simulink model "hexapod2"  (R2015a)
settings: Solver=ode23tb  StartTime=0.0  StopTime=10  FixedStep=0.0001  MaxStep=0.01  RelTol=1e-4  AbsTol=1e-5
values from neighbouring files (symbols this model uses):
  bH = 1    [runFirst.m]
  C = CM + CL/n^2    (= 0.0001377500155)    [runFirst.m]
  d1 = 0    [runFirst.m]    (also in runFirst2.m)
  d2 = -4.61    [runFirst.m]    (also in runFirst2.m = 0)
  J = JM + JL/n^2    (= 0.008455500031)    [runFirst.m]
  Ka = 12    [runFirst.m]
  Kb = 0.00867    [runFirst.m]
  Ke = 1    [runFirst.m]
  Km = 4.375    [runFirst.m]
  L = 0.0006    [runFirst.m]
  L1 = 3.64    [runFirst.m]    (also in runFirst2.m = 3.4)
  L2 = 5.72    [runFirst.m]    (also in runFirst2.m = 8.7)
  L3 = 12.46    [runFirst.m]    (also in runFirst2.m = 12.73)
  n = 254    [runFirst.m]
  R = 1.4    [runFirst.m]
undefined symbols (not defined in the file or in its folder): bLb, bLs, X, Y, Z
libraries: sm_lib x108, nesl_utility x43, simulink x24, Contact_Forces_Lib x7, roblocks x2
(part 4 of 5)

== system hexapod2/Hexapod/Leg4/Link3 ==
  Reference Frame : sm_lib/Frames and Transforms/Reference Frame  BlockFunction=simmechanics.library.frames_transforms.reference_frame
  Rigid Transform : sm_lib/Frames and Transforms/Rigid Transform  TranslationMethod=StandardAxis  TranslationLengthUnit=cm  TranslationStandardAxis=+X  TranslationStandardOffset=L/2  TranslationCartesianOffset=[0 0 0]  TranslationROffset=0  TranslationROffsetUnits=m  TranslationZOffset=0  TranslationZOffsetUnits=m  TranslationThetaOffset=0  TranslationThetaOffsetUnits=deg  RotationMethod=None  RotationAngleUnits=deg  RotationStandardAxis=+X  RotationAngle=Xangle  RotationArbitraryAxis=[0 0 1]  FollAlignAxisA=+X  BaseAlignAxisA=+Y  FollAlignAxisB=+Y  BaseAlignAxisB=+Z  RotationMatrix=[1 0 0; 0 1 0; 0 0 1]  BlockFunction=simmechanics.library.frames_transforms.rigid_transform
  Rigid Transform1 : sm_lib/Frames and Transforms/Rigid Transform  TranslationMethod=StandardAxis  TranslationLengthUnit=cm  TranslationStandardAxis=-X  TranslationStandardOffset=L/2  TranslationCartesianOffset=[0 0 0]  TranslationROffset=0  TranslationROffsetUnits=m  TranslationZOffset=0  TranslationZOffsetUnits=m  TranslationThetaOffset=0  TranslationThetaOffsetUnits=deg  RotationMethod=None  RotationAngleUnits=deg  RotationStandardAxis=+Z  RotationAngle=0.0  RotationArbitraryAxis=[0 0 1]  FollAlignAxisA=+X  BaseAlignAxisA=+Y  FollAlignAxisB=+Y  BaseAlignAxisB=+Z  RotationMatrix=[1 0 0; 0 1 0; 0 0 1]  BlockFunction=simmechanics.library.frames_transforms.rigid_transform
  Solid : sm_lib/Body Elements/Solid  InertiaType=PointMass  Mass=m  MassUnits=kg  CenterOfMass=[0 0 0]  CenterOfMassUnits=m  MomentsOfInertia=[1 1 1]  MomentsOfInertiaUnits=kg*m^2  ProductsOfInertia=[0 0 0]  ProductsOfInertiaUnits=kg*m^2  DensityBased=off  Density=1  DensityUnits=kg/(m^3)  GraphicType=FromGeometry  MarkerShape=Sphere  MarkerSize=10  MarkerSizeUnits=m  GraphicVisPropType=SimpleVisualProperties  GraphicDiffuseColor=rgb  GraphicSpecularColor=[0.5 0.5 0.5 1.0]  GraphicAmbientColor=[0.15 0.15 0.15 1.0]  GraphicEmissiveColor=[0.0 0.0 0.0 1.0]  GraphicShininess=75  GraphicOpacity=1.0  GeometryShape=Brick  RectangleSize=[1 1]  RectangleSizeUnits=m  BrickDimensions=[L W H]  BrickDimensionUnits=cm  CylinderRadius=1  CylinderRadiusUnits=m  CylinderLength=1  CylinderLengthUnits=m  SphereRadius=1  SphereRadiusUnits=m  EllipsoidRadii=[1 1 1]  EllipsoidRadiiUnits=m  ExtrusionCrossSection=[1 1; -1 1; -1 -1; 1 -1]  ExtrusionCrossSectionUnits=m  ExtrusionLength=1  ExtrusionLengthUnits=m  PolygonNumSides=3  PolygonOuterRadius=1  PolygonOuterRadiusUnits=m  ExtGeomFileType=STL  ExtGeomFileUnits=m  RevolutionCrossSection=[1 1; 1 -1; 2 -1; 2 1]  RevolutionCrossSectionUnits=m  RevolutionExtent=Full  RevolutionAngle=180  RevolutionAngleUnits=deg  BlockFunction=simmechanics.library.body_elements.solid
  Conn1 : PMIOPort  Port=1  Side=Left
  Conn2 : PMIOPort  Port=2  Side=Right
  connections:
  Reference Frame/RConn1 -- Solid/RConn1 -- Rigid Transform/LConn1 -- Rigid Transform1/LConn1
  Rigid Transform/RConn1 -- Conn2/RConn1
  Rigid Transform1/RConn1 -- Conn1/RConn1

== system hexapod2/Hexapod/Leg4/Servo ==
  note: ThetaRef
  note: e
  note: Vref
  thetaRef : Inport
  PID : Subsystem
  Sum : Sum  Inputs=|+-
  Thet : Scope
      settings: TimeRange=10  YMin=0  YMax=21
  w : Scope
      settings: SaveName=ScopeData2
  wd : Scope
      settings: SaveName=ScopeData3
  Двигатель : Subsystem
  Заданный угол : Gain
  Энкодер : Gain  Gain=Ke
  theta : Outport
  wires:
  thetaRef/1 -> Заданный угол/1
  Двигатель/3(Ускорение) -> wd/1
  PID/1(Out1) -> Двигатель/1(Заданный угол)
  Двигатель/1(Угол) -> Энкодер/1, Thet/1, theta/1
  Энкодер/1 -> Sum/2
  Sum/1 -> PID/1(In1)
  Заданный угол/1 -> Sum/1
  Двигатель/2(Скорость) -> w/1

== system hexapod2/Hexapod/Leg4/Servo1 ==
  note: Vref
  note: e
  note: ThetaRef
  thetaRef : Inport
  PID : Subsystem
  Sum : Sum  Inputs=|+-
  Thet : Scope
      settings: TimeRange=10  YMin=0  YMax=21
  w : Scope
      settings: SaveName=ScopeData2
  wd : Scope
      settings: SaveName=ScopeData3
  Двигатель : Subsystem
  Заданный угол : Gain
  Энкодер : Gain  Gain=Ke
  theta : Outport
  wires:
  Двигатель/2(Скорость) -> w/1
  Заданный угол/1 -> Sum/1
  Sum/1 -> PID/1(In1)
  Энкодер/1 -> Sum/2
  Двигатель/1(Угол) -> theta/1, Thet/1, Энкодер/1
  PID/1(Out1) -> Двигатель/1(Заданный угол)
  Двигатель/3(Ускорение) -> wd/1
  thetaRef/1 -> Заданный угол/1

== system hexapod2/Hexapod/Leg4/Servo2 ==
  note: ThetaRef
  note: e
  note: Vref
  thetaRef : Inport
  PID : Subsystem
  Sum : Sum  Inputs=|+-
  Thet : Scope
      settings: TimeRange=10  YMin=0  YMax=21
  w : Scope
      settings: SaveName=ScopeData2
  wd : Scope
      settings: SaveName=ScopeData3
  Двигатель : Subsystem
  Заданный угол : Gain
  Энкодер : Gain  Gain=Ke
  theta : Outport
  wires:
  thetaRef/1 -> Заданный угол/1
  Двигатель/3(Ускорение) -> wd/1
  PID/1(Out1) -> Двигатель/1(Заданный угол)
  Двигатель/1(Угол) -> Энкодер/1, Thet/1, theta/1
  Энкодер/1 -> Sum/2
  Sum/1 -> PID/1(In1)
  Заданный угол/1 -> Sum/1
  Двигатель/2(Скорость) -> w/1

== system hexapod2/Hexapod/Leg5/Link1 ==
  Reference Frame : sm_lib/Frames and Transforms/Reference Frame  BlockFunction=simmechanics.library.frames_transforms.reference_frame
  Rigid Transform : sm_lib/Frames and Transforms/Rigid Transform  TranslationMethod=Cartesian  TranslationLengthUnit=cm  TranslationStandardAxis=+X  TranslationStandardOffset=L/2  TranslationCartesianOffset=[L/2 0 -2.3]  TranslationROffset=0  TranslationROffsetUnits=m  TranslationZOffset=0  TranslationZOffsetUnits=m  TranslationThetaOffset=0  TranslationThetaOffsetUnits=deg  RotationMethod=StandardAxis  RotationAngleUnits=deg  RotationStandardAxis=+X  RotationAngle=Xangle  RotationArbitraryAxis=[0 0 1]  FollAlignAxisA=+X  BaseAlignAxisA=+Y  FollAlignAxisB=+Y  BaseAlignAxisB=+Z  RotationMatrix=[1 0 0; 0 1 0; 0 0 1]  BlockFunction=simmechanics.library.frames_transforms.rigid_transform
  Rigid Transform1 : sm_lib/Frames and Transforms/Rigid Transform  TranslationMethod=StandardAxis  TranslationLengthUnit=cm  TranslationStandardAxis=-X  TranslationStandardOffset=L/2  TranslationCartesianOffset=[0 0 0]  TranslationROffset=0  TranslationROffsetUnits=m  TranslationZOffset=0  TranslationZOffsetUnits=m  TranslationThetaOffset=0  TranslationThetaOffsetUnits=deg  RotationMethod=None  RotationAngleUnits=deg  RotationStandardAxis=+Z  RotationAngle=0.0  RotationArbitraryAxis=[0 0 1]  FollAlignAxisA=+X  BaseAlignAxisA=+Y  FollAlignAxisB=+Y  BaseAlignAxisB=+Z  RotationMatrix=[1 0 0; 0 1 0; 0 0 1]  BlockFunction=simmechanics.library.frames_transforms.rigid_transform
  Solid : sm_lib/Body Elements/Solid  InertiaType=PointMass  Mass=m  MassUnits=kg  CenterOfMass=[0 0 0]  CenterOfMassUnits=m  MomentsOfInertia=[1 1 1]  MomentsOfInertiaUnits=kg*m^2  ProductsOfInertia=[0 0 0]  ProductsOfInertiaUnits=kg*m^2  DensityBased=off  Density=1  DensityUnits=kg/(m^3)  GraphicType=FromGeometry  MarkerShape=Sphere  MarkerSize=10  MarkerSizeUnits=m  GraphicVisPropType=SimpleVisualProperties  GraphicDiffuseColor=rgb  GraphicSpecularColor=[0.5 0.5 0.5 1.0]  GraphicAmbientColor=[0.15 0.15 0.15 1.0]  GraphicEmissiveColor=[0.0 0.0 0.0 1.0]  GraphicShininess=75  GraphicOpacity=1.0  GeometryShape=Brick  RectangleSize=[1 1]  RectangleSizeUnits=m  BrickDimensions=[L W H]  BrickDimensionUnits=cm  CylinderRadius=1  CylinderRadiusUnits=m  CylinderLength=1  CylinderLengthUnits=m  SphereRadius=1  SphereRadiusUnits=m  EllipsoidRadii=[1 1 1]  EllipsoidRadiiUnits=m  ExtrusionCrossSection=[1 1; -1 1; -1 -1; 1 -1]  ExtrusionCrossSectionUnits=m  ExtrusionLength=1  ExtrusionLengthUnits=m  PolygonNumSides=3  PolygonOuterRadius=1  PolygonOuterRadiusUnits=m  ExtGeomFileType=STL  ExtGeomFileUnits=m  RevolutionCrossSection=[1 1; 1 -1; 2 -1; 2 1]  RevolutionCrossSectionUnits=m  RevolutionExtent=Full  RevolutionAngle=180  RevolutionAngleUnits=deg  BlockFunction=simmechanics.library.body_elements.solid
  Conn1 : PMIOPort  Port=1  Side=Left
  Conn2 : PMIOPort  Port=2  Side=Right
  connections:
  Rigid Transform1/RConn1 -- Conn1/RConn1
  Rigid Transform/RConn1 -- Conn2/RConn1
  Rigid Transform1/LConn1 -- Rigid Transform/LConn1 -- Solid/RConn1 -- Reference Frame/RConn1

== system hexapod2/Hexapod/Leg5/Link2 ==
  Reference Frame : sm_lib/Frames and Transforms/Reference Frame  BlockFunction=simmechanics.library.frames_transforms.reference_frame
  Rigid Transform : sm_lib/Frames and Transforms/Rigid Transform  TranslationMethod=StandardAxis  TranslationLengthUnit=cm  TranslationStandardAxis=+X  TranslationStandardOffset=L/2  TranslationCartesianOffset=[0 0 0]  TranslationROffset=0  TranslationROffsetUnits=m  TranslationZOffset=0  TranslationZOffsetUnits=m  TranslationThetaOffset=0  TranslationThetaOffsetUnits=deg  RotationMethod=StandardAxis  RotationAngleUnits=deg  RotationStandardAxis=+X  RotationAngle=Xangle  RotationArbitraryAxis=[0 0 1]  FollAlignAxisA=+X  BaseAlignAxisA=+Y  FollAlignAxisB=+Y  BaseAlignAxisB=+Z  RotationMatrix=[1 0 0; 0 1 0; 0 0 1]  BlockFunction=simmechanics.library.frames_transforms.rigid_transform
  Rigid Transform1 : sm_lib/Frames and Transforms/Rigid Transform  TranslationMethod=StandardAxis  TranslationLengthUnit=cm  TranslationStandardAxis=-X  TranslationStandardOffset=L/2  TranslationCartesianOffset=[0 0 0]  TranslationROffset=0  TranslationROffsetUnits=m  TranslationZOffset=0  TranslationZOffsetUnits=m  TranslationThetaOffset=0  TranslationThetaOffsetUnits=deg  RotationMethod=None  RotationAngleUnits=deg  RotationStandardAxis=+Z  RotationAngle=0.0  RotationArbitraryAxis=[0 0 1]  FollAlignAxisA=+X  BaseAlignAxisA=+Y  FollAlignAxisB=+Y  BaseAlignAxisB=+Z  RotationMatrix=[1 0 0; 0 1 0; 0 0 1]  BlockFunction=simmechanics.library.frames_transforms.rigid_transform
  Solid : sm_lib/Body Elements/Solid  InertiaType=PointMass  Mass=m  MassUnits=kg  CenterOfMass=[0 0 0]  CenterOfMassUnits=m  MomentsOfInertia=[1 1 1]  MomentsOfInertiaUnits=kg*m^2  ProductsOfInertia=[0 0 0]  ProductsOfInertiaUnits=kg*m^2  DensityBased=off  Density=1  DensityUnits=kg/(m^3)  GraphicType=FromGeometry  MarkerShape=Sphere  MarkerSize=10  MarkerSizeUnits=m  GraphicVisPropType=SimpleVisualProperties  GraphicDiffuseColor=rgb  GraphicSpecularColor=[0.5 0.5 0.5 1.0]  GraphicAmbientColor=[0.15 0.15 0.15 1.0]  GraphicEmissiveColor=[0.0 0.0 0.0 1.0]  GraphicShininess=75  GraphicOpacity=1.0  GeometryShape=Brick  RectangleSize=[1 1]  RectangleSizeUnits=m  BrickDimensions=[L W H]  BrickDimensionUnits=cm  CylinderRadius=1  CylinderRadiusUnits=m  CylinderLength=1  CylinderLengthUnits=m  SphereRadius=1  SphereRadiusUnits=m  EllipsoidRadii=[1 1 1]  EllipsoidRadiiUnits=m  ExtrusionCrossSection=[1 1; -1 1; -1 -1; 1 -1]  ExtrusionCrossSectionUnits=m  ExtrusionLength=1  ExtrusionLengthUnits=m  PolygonNumSides=3  PolygonOuterRadius=1  PolygonOuterRadiusUnits=m  ExtGeomFileType=STL  ExtGeomFileUnits=m  RevolutionCrossSection=[1 1; 1 -1; 2 -1; 2 1]  RevolutionCrossSectionUnits=m  RevolutionExtent=Full  RevolutionAngle=180  RevolutionAngleUnits=deg  BlockFunction=simmechanics.library.body_elements.solid
  Conn1 : PMIOPort  Port=1  Side=Left
  Conn2 : PMIOPort  Port=2  Side=Right
  connections:
  Reference Frame/RConn1 -- Solid/RConn1 -- Rigid Transform/LConn1 -- Rigid Transform1/LConn1
  Rigid Transform/RConn1 -- Conn2/RConn1
  Rigid Transform1/RConn1 -- Conn1/RConn1

== system hexapod2/Hexapod/Leg5/Link3 ==
  Reference Frame : sm_lib/Frames and Transforms/Reference Frame  BlockFunction=simmechanics.library.frames_transforms.reference_frame
  Rigid Transform : sm_lib/Frames and Transforms/Rigid Transform  TranslationMethod=StandardAxis  TranslationLengthUnit=cm  TranslationStandardAxis=+X  TranslationStandardOffset=L/2  TranslationCartesianOffset=[0 0 0]  TranslationROffset=0  TranslationROffsetUnits=m  TranslationZOffset=0  TranslationZOffsetUnits=m  TranslationThetaOffset=0  TranslationThetaOffsetUnits=deg  RotationMethod=None  RotationAngleUnits=deg  RotationStandardAxis=+X  RotationAngle=Xangle  RotationArbitraryAxis=[0 0 1]  FollAlignAxisA=+X  BaseAlignAxisA=+Y  FollAlignAxisB=+Y  BaseAlignAxisB=+Z  RotationMatrix=[1 0 0; 0 1 0; 0 0 1]  BlockFunction=simmechanics.library.frames_transforms.rigid_transform
  Rigid Transform1 : sm_lib/Frames and Transforms/Rigid Transform  TranslationMethod=StandardAxis  TranslationLengthUnit=cm  TranslationStandardAxis=-X  TranslationStandardOffset=L/2  TranslationCartesianOffset=[0 0 0]  TranslationROffset=0  TranslationROffsetUnits=m  TranslationZOffset=0  TranslationZOffsetUnits=m  TranslationThetaOffset=0  TranslationThetaOffsetUnits=deg  RotationMethod=None  RotationAngleUnits=deg  RotationStandardAxis=+Z  RotationAngle=0.0  RotationArbitraryAxis=[0 0 1]  FollAlignAxisA=+X  BaseAlignAxisA=+Y  FollAlignAxisB=+Y  BaseAlignAxisB=+Z  RotationMatrix=[1 0 0; 0 1 0; 0 0 1]  BlockFunction=simmechanics.library.frames_transforms.rigid_transform
  Solid : sm_lib/Body Elements/Solid  InertiaType=PointMass  Mass=m  MassUnits=kg  CenterOfMass=[0 0 0]  CenterOfMassUnits=m  MomentsOfInertia=[1 1 1]  MomentsOfInertiaUnits=kg*m^2  ProductsOfInertia=[0 0 0]  ProductsOfInertiaUnits=kg*m^2  DensityBased=off  Density=1  DensityUnits=kg/(m^3)  GraphicType=FromGeometry  MarkerShape=Sphere  MarkerSize=10  MarkerSizeUnits=m  GraphicVisPropType=SimpleVisualProperties  GraphicDiffuseColor=rgb  GraphicSpecularColor=[0.5 0.5 0.5 1.0]  GraphicAmbientColor=[0.15 0.15 0.15 1.0]  GraphicEmissiveColor=[0.0 0.0 0.0 1.0]  GraphicShininess=75  GraphicOpacity=1.0  GeometryShape=Brick  RectangleSize=[1 1]  RectangleSizeUnits=m  BrickDimensions=[L W H]  BrickDimensionUnits=cm  CylinderRadius=1  CylinderRadiusUnits=m  CylinderLength=1  CylinderLengthUnits=m  SphereRadius=1  SphereRadiusUnits=m  EllipsoidRadii=[1 1 1]  EllipsoidRadiiUnits=m  ExtrusionCrossSection=[1 1; -1 1; -1 -1; 1 -1]  ExtrusionCrossSectionUnits=m  ExtrusionLength=1  ExtrusionLengthUnits=m  PolygonNumSides=3  PolygonOuterRadius=1  PolygonOuterRadiusUnits=m  ExtGeomFileType=STL  ExtGeomFileUnits=m  RevolutionCrossSection=[1 1; 1 -1; 2 -1; 2 1]  RevolutionCrossSectionUnits=m  RevolutionExtent=Full  RevolutionAngle=180  RevolutionAngleUnits=deg  BlockFunction=simmechanics.library.body_elements.solid
  Conn1 : PMIOPort  Port=1  Side=Left
  Conn2 : PMIOPort  Port=2  Side=Right
  connections:
  Rigid Transform1/RConn1 -- Conn1/RConn1
  Rigid Transform/RConn1 -- Conn2/RConn1
  Rigid Transform1/LConn1 -- Rigid Transform/LConn1 -- Solid/RConn1 -- Reference Frame/RConn1

== system hexapod2/Hexapod/Leg5/Servo ==
  note: Vref
  note: e
  note: ThetaRef
  thetaRef : Inport
  PID : Subsystem
  Sum : Sum  Inputs=|+-
  Thet : Scope
      settings: TimeRange=10  YMin=0  YMax=21
  w : Scope
      settings: SaveName=ScopeData2
  wd : Scope
      settings: SaveName=ScopeData3
  Двигатель : Subsystem
  Заданный угол : Gain
  Энкодер : Gain  Gain=Ke
  theta : Outport
  wires:
  Двигатель/2(Скорость) -> w/1
  Заданный угол/1 -> Sum/1
  Sum/1 -> PID/1(In1)
  Энкодер/1 -> Sum/2
  Двигатель/1(Угол) -> theta/1, Thet/1, Энкодер/1
  PID/1(Out1) -> Двигатель/1(Заданный угол)
  Двигатель/3(Ускорение) -> wd/1
  thetaRef/1 -> Заданный угол/1

== system hexapod2/Hexapod/Leg5/Servo1 ==
  note: ThetaRef
  note: e
  note: Vref
  thetaRef : Inport
  PID : Subsystem
  Sum : Sum  Inputs=|+-
  Thet : Scope
      settings: TimeRange=10  YMin=0  YMax=21
  w : Scope
      settings: SaveName=ScopeData2
  wd : Scope
      settings: SaveName=ScopeData3
  Двигатель : Subsystem
  Заданный угол : Gain
  Энкодер : Gain  Gain=Ke
  theta : Outport
  wires:
  thetaRef/1 -> Заданный угол/1
  Двигатель/3(Ускорение) -> wd/1
  PID/1(Out1) -> Двигатель/1(Заданный угол)
  Двигатель/1(Угол) -> Энкодер/1, Thet/1, theta/1
  Энкодер/1 -> Sum/2
  Sum/1 -> PID/1(In1)
  Заданный угол/1 -> Sum/1
  Двигатель/2(Скорость) -> w/1

== system hexapod2/Hexapod/Leg5/Servo2 ==
  note: Vref
  note: e
  note: ThetaRef
  thetaRef : Inport
  PID : Subsystem
  Sum : Sum  Inputs=|+-
  Thet : Scope
      settings: TimeRange=10  YMin=0  YMax=21
  w : Scope
      settings: SaveName=ScopeData2
  wd : Scope
      settings: SaveName=ScopeData3
  Двигатель : Subsystem
  Заданный угол : Gain
  Энкодер : Gain  Gain=Ke
  theta : Outport
  wires:
  Двигатель/2(Скорость) -> w/1
  Заданный угол/1 -> Sum/1
  Sum/1 -> PID/1(In1)
  Энкодер/1 -> Sum/2
  Двигатель/1(Угол) -> theta/1, Thet/1, Энкодер/1
  PID/1(Out1) -> Двигатель/1(Заданный угол)
  Двигатель/3(Ускорение) -> wd/1
  thetaRef/1 -> Заданный угол/1

== system hexapod2/Hexapod/Leg6/Link1 ==
  Reference Frame : sm_lib/Frames and Transforms/Reference Frame  BlockFunction=simmechanics.library.frames_transforms.reference_frame
  Rigid Transform : sm_lib/Frames and Transforms/Rigid Transform  TranslationMethod=Cartesian  TranslationLengthUnit=cm  TranslationStandardAxis=+X  TranslationStandardOffset=L/2  TranslationCartesianOffset=[L/2 0 -2.3]  TranslationROffset=0  TranslationROffsetUnits=m  TranslationZOffset=0  TranslationZOffsetUnits=m  TranslationThetaOffset=0  TranslationThetaOffsetUnits=deg  RotationMethod=StandardAxis  RotationAngleUnits=deg  RotationStandardAxis=+X  RotationAngle=Xangle  RotationArbitraryAxis=[0 0 1]  FollAlignAxisA=+X  BaseAlignAxisA=+Y  FollAlignAxisB=+Y  BaseAlignAxisB=+Z  RotationMatrix=[1 0 0; 0 1 0; 0 0 1]  BlockFunction=simmechanics.library.frames_transforms.rigid_transform
  Rigid Transform1 : sm_lib/Frames and Transforms/Rigid Transform  TranslationMethod=StandardAxis  TranslationLengthUnit=cm  TranslationStandardAxis=-X  TranslationStandardOffset=L/2  TranslationCartesianOffset=[0 0 0]  TranslationROffset=0  TranslationROffsetUnits=m  TranslationZOffset=0  TranslationZOffsetUnits=m  TranslationThetaOffset=0  TranslationThetaOffsetUnits=deg  RotationMethod=None  RotationAngleUnits=deg  RotationStandardAxis=+Z  RotationAngle=0.0  RotationArbitraryAxis=[0 0 1]  FollAlignAxisA=+X  BaseAlignAxisA=+Y  FollAlignAxisB=+Y  BaseAlignAxisB=+Z  RotationMatrix=[1 0 0; 0 1 0; 0 0 1]  BlockFunction=simmechanics.library.frames_transforms.rigid_transform
  Solid : sm_lib/Body Elements/Solid  InertiaType=PointMass  Mass=m  MassUnits=kg  CenterOfMass=[0 0 0]  CenterOfMassUnits=m  MomentsOfInertia=[1 1 1]  MomentsOfInertiaUnits=kg*m^2  ProductsOfInertia=[0 0 0]  ProductsOfInertiaUnits=kg*m^2  DensityBased=off  Density=1  DensityUnits=kg/(m^3)  GraphicType=FromGeometry  MarkerShape=Sphere  MarkerSize=10  MarkerSizeUnits=m  GraphicVisPropType=SimpleVisualProperties  GraphicDiffuseColor=rgb  GraphicSpecularColor=[0.5 0.5 0.5 1.0]  GraphicAmbientColor=[0.15 0.15 0.15 1.0]  GraphicEmissiveColor=[0.0 0.0 0.0 1.0]  GraphicShininess=75  GraphicOpacity=1.0  GeometryShape=Brick  RectangleSize=[1 1]  RectangleSizeUnits=m  BrickDimensions=[L W H]  BrickDimensionUnits=cm  CylinderRadius=1  CylinderRadiusUnits=m  CylinderLength=1  CylinderLengthUnits=m  SphereRadius=1  SphereRadiusUnits=m  EllipsoidRadii=[1 1 1]  EllipsoidRadiiUnits=m  ExtrusionCrossSection=[1 1; -1 1; -1 -1; 1 -1]  ExtrusionCrossSectionUnits=m  ExtrusionLength=1  ExtrusionLengthUnits=m  PolygonNumSides=3  PolygonOuterRadius=1  PolygonOuterRadiusUnits=m  ExtGeomFileType=STL  ExtGeomFileUnits=m  RevolutionCrossSection=[1 1; 1 -1; 2 -1; 2 1]  RevolutionCrossSectionUnits=m  RevolutionExtent=Full  RevolutionAngle=180  RevolutionAngleUnits=deg  BlockFunction=simmechanics.library.body_elements.solid
  Conn1 : PMIOPort  Port=1  Side=Left
  Conn2 : PMIOPort  Port=2  Side=Right
  connections:
  Reference Frame/RConn1 -- Solid/RConn1 -- Rigid Transform/LConn1 -- Rigid Transform1/LConn1
  Rigid Transform/RConn1 -- Conn2/RConn1
  Rigid Transform1/RConn1 -- Conn1/RConn1

== system hexapod2/Hexapod/Leg6/Link2 ==
  Reference Frame : sm_lib/Frames and Transforms/Reference Frame  BlockFunction=simmechanics.library.frames_transforms.reference_frame
  Rigid Transform : sm_lib/Frames and Transforms/Rigid Transform  TranslationMethod=StandardAxis  TranslationLengthUnit=cm  TranslationStandardAxis=+X  TranslationStandardOffset=L/2  TranslationCartesianOffset=[0 0 0]  TranslationROffset=0  TranslationROffsetUnits=m  TranslationZOffset=0  TranslationZOffsetUnits=m  TranslationThetaOffset=0  TranslationThetaOffsetUnits=deg  RotationMethod=StandardAxis  RotationAngleUnits=deg  RotationStandardAxis=+X  RotationAngle=Xangle  RotationArbitraryAxis=[0 0 1]  FollAlignAxisA=+X  BaseAlignAxisA=+Y  FollAlignAxisB=+Y  BaseAlignAxisB=+Z  RotationMatrix=[1 0 0; 0 1 0; 0 0 1]  BlockFunction=simmechanics.library.frames_transforms.rigid_transform
  Rigid Transform1 : sm_lib/Frames and Transforms/Rigid Transform  TranslationMethod=StandardAxis  TranslationLengthUnit=cm  TranslationStandardAxis=-X  TranslationStandardOffset=L/2  TranslationCartesianOffset=[0 0 0]  TranslationROffset=0  TranslationROffsetUnits=m  TranslationZOffset=0  TranslationZOffsetUnits=m  TranslationThetaOffset=0  TranslationThetaOffsetUnits=deg  RotationMethod=None  RotationAngleUnits=deg  RotationStandardAxis=+Z  RotationAngle=0.0  RotationArbitraryAxis=[0 0 1]  FollAlignAxisA=+X  BaseAlignAxisA=+Y  FollAlignAxisB=+Y  BaseAlignAxisB=+Z  RotationMatrix=[1 0 0; 0 1 0; 0 0 1]  BlockFunction=simmechanics.library.frames_transforms.rigid_transform
  Solid : sm_lib/Body Elements/Solid  InertiaType=PointMass  Mass=m  MassUnits=kg  CenterOfMass=[0 0 0]  CenterOfMassUnits=m  MomentsOfInertia=[1 1 1]  MomentsOfInertiaUnits=kg*m^2  ProductsOfInertia=[0 0 0]  ProductsOfInertiaUnits=kg*m^2  DensityBased=off  Density=1  DensityUnits=kg/(m^3)  GraphicType=FromGeometry  MarkerShape=Sphere  MarkerSize=10  MarkerSizeUnits=m  GraphicVisPropType=SimpleVisualProperties  GraphicDiffuseColor=rgb  GraphicSpecularColor=[0.5 0.5 0.5 1.0]  GraphicAmbientColor=[0.15 0.15 0.15 1.0]  GraphicEmissiveColor=[0.0 0.0 0.0 1.0]  GraphicShininess=75  GraphicOpacity=1.0  GeometryShape=Brick  RectangleSize=[1 1]  RectangleSizeUnits=m  BrickDimensions=[L W H]  BrickDimensionUnits=cm  CylinderRadius=1  CylinderRadiusUnits=m  CylinderLength=1  CylinderLengthUnits=m  SphereRadius=1  SphereRadiusUnits=m  EllipsoidRadii=[1 1 1]  EllipsoidRadiiUnits=m  ExtrusionCrossSection=[1 1; -1 1; -1 -1; 1 -1]  ExtrusionCrossSectionUnits=m  ExtrusionLength=1  ExtrusionLengthUnits=m  PolygonNumSides=3  PolygonOuterRadius=1  PolygonOuterRadiusUnits=m  ExtGeomFileType=STL  ExtGeomFileUnits=m  RevolutionCrossSection=[1 1; 1 -1; 2 -1; 2 1]  RevolutionCrossSectionUnits=m  RevolutionExtent=Full  RevolutionAngle=180  RevolutionAngleUnits=deg  BlockFunction=simmechanics.library.body_elements.solid
  Conn1 : PMIOPort  Port=1  Side=Left
  Conn2 : PMIOPort  Port=2  Side=Right
  connections:
  Rigid Transform1/RConn1 -- Conn1/RConn1
  Rigid Transform/RConn1 -- Conn2/RConn1
  Rigid Transform1/LConn1 -- Rigid Transform/LConn1 -- Solid/RConn1 -- Reference Frame/RConn1

== system hexapod2/Hexapod/Leg6/Link3 ==
  Reference Frame : sm_lib/Frames and Transforms/Reference Frame  BlockFunction=simmechanics.library.frames_transforms.reference_frame
  Rigid Transform : sm_lib/Frames and Transforms/Rigid Transform  TranslationMethod=StandardAxis  TranslationLengthUnit=cm  TranslationStandardAxis=+X  TranslationStandardOffset=L/2  TranslationCartesianOffset=[0 0 0]  TranslationROffset=0  TranslationROffsetUnits=m  TranslationZOffset=0  TranslationZOffsetUnits=m  TranslationThetaOffset=0  TranslationThetaOffsetUnits=deg  RotationMethod=None  RotationAngleUnits=deg  RotationStandardAxis=+X  RotationAngle=Xangle  RotationArbitraryAxis=[0 0 1]  FollAlignAxisA=+X  BaseAlignAxisA=+Y  FollAlignAxisB=+Y  BaseAlignAxisB=+Z  RotationMatrix=[1 0 0; 0 1 0; 0 0 1]  BlockFunction=simmechanics.library.frames_transforms.rigid_transform
  Rigid Transform1 : sm_lib/Frames and Transforms/Rigid Transform  TranslationMethod=StandardAxis  TranslationLengthUnit=cm  TranslationStandardAxis=-X  TranslationStandardOffset=L/2  TranslationCartesianOffset=[0 0 0]  TranslationROffset=0  TranslationROffsetUnits=m  TranslationZOffset=0  TranslationZOffsetUnits=m  TranslationThetaOffset=0  TranslationThetaOffsetUnits=deg  RotationMethod=None  RotationAngleUnits=deg  RotationStandardAxis=+Z  RotationAngle=0.0  RotationArbitraryAxis=[0 0 1]  FollAlignAxisA=+X  BaseAlignAxisA=+Y  FollAlignAxisB=+Y  BaseAlignAxisB=+Z  RotationMatrix=[1 0 0; 0 1 0; 0 0 1]  BlockFunction=simmechanics.library.frames_transforms.rigid_transform
  Solid : sm_lib/Body Elements/Solid  InertiaType=PointMass  Mass=m  MassUnits=kg  CenterOfMass=[0 0 0]  CenterOfMassUnits=m  MomentsOfInertia=[1 1 1]  MomentsOfInertiaUnits=kg*m^2  ProductsOfInertia=[0 0 0]  ProductsOfInertiaUnits=kg*m^2  DensityBased=off  Density=1  DensityUnits=kg/(m^3)  GraphicType=FromGeometry  MarkerShape=Sphere  MarkerSize=10  MarkerSizeUnits=m  GraphicVisPropType=SimpleVisualProperties  GraphicDiffuseColor=rgb  GraphicSpecularColor=[0.5 0.5 0.5 1.0]  GraphicAmbientColor=[0.15 0.15 0.15 1.0]  GraphicEmissiveColor=[0.0 0.0 0.0 1.0]  GraphicShininess=75  GraphicOpacity=1.0  GeometryShape=Brick  RectangleSize=[1 1]  RectangleSizeUnits=m  BrickDimensions=[L W H]  BrickDimensionUnits=cm  CylinderRadius=1  CylinderRadiusUnits=m  CylinderLength=1  CylinderLengthUnits=m  SphereRadius=1  SphereRadiusUnits=m  EllipsoidRadii=[1 1 1]  EllipsoidRadiiUnits=m  ExtrusionCrossSection=[1 1; -1 1; -1 -1; 1 -1]  ExtrusionCrossSectionUnits=m  ExtrusionLength=1  ExtrusionLengthUnits=m  PolygonNumSides=3  PolygonOuterRadius=1  PolygonOuterRadiusUnits=m  ExtGeomFileType=STL  ExtGeomFileUnits=m  RevolutionCrossSection=[1 1; 1 -1; 2 -1; 2 1]  RevolutionCrossSectionUnits=m  RevolutionExtent=Full  RevolutionAngle=180  RevolutionAngleUnits=deg  BlockFunction=simmechanics.library.body_elements.solid
  Conn1 : PMIOPort  Port=1  Side=Left
  Conn2 : PMIOPort  Port=2  Side=Right
  connections:
  Reference Frame/RConn1 -- Solid/RConn1 -- Rigid Transform/LConn1 -- Rigid Transform1/LConn1
  Rigid Transform/RConn1 -- Conn2/RConn1
  Rigid Transform1/RConn1 -- Conn1/RConn1

== system hexapod2/Hexapod/Leg6/Servo ==
  note: ThetaRef
  note: e
  note: Vref
  thetaRef : Inport
  PID : Subsystem
  Sum : Sum  Inputs=|+-
  Thet : Scope
      settings: TimeRange=10  YMin=0  YMax=21
  w : Scope
      settings: SaveName=ScopeData2
  wd : Scope
      settings: SaveName=ScopeData3
  Двигатель : Subsystem
  Заданный угол : Gain
  Энкодер : Gain  Gain=Ke
  theta : Outport
  wires:
  thetaRef/1 -> Заданный угол/1
  Двигатель/3(Ускорение) -> wd/1
  PID/1(Out1) -> Двигатель/1(Заданный угол)
  Двигатель/1(Угол) -> Энкодер/1, Thet/1, theta/1
  Энкодер/1 -> Sum/2
  Sum/1 -> PID/1(In1)
  Заданный угол/1 -> Sum/1
  Двигатель/2(Скорость) -> w/1

== system hexapod2/Hexapod/Leg6/Servo1 ==
  note: Vref
  note: e
  note: ThetaRef
  thetaRef : Inport
  PID : Subsystem
  Sum : Sum  Inputs=|+-
  Thet : Scope
      settings: TimeRange=10  YMin=0  YMax=21
  w : Scope
      settings: SaveName=ScopeData2
  wd : Scope
      settings: SaveName=ScopeData3
  Двигатель : Subsystem
  Заданный угол : Gain
  Энкодер : Gain  Gain=Ke
  theta : Outport
  wires:
  Двигатель/2(Скорость) -> w/1
  Заданный угол/1 -> Sum/1
  Sum/1 -> PID/1(In1)
  Энкодер/1 -> Sum/2
  Двигатель/1(Угол) -> theta/1, Thet/1, Энкодер/1
  PID/1(Out1) -> Двигатель/1(Заданный угол)
  Двигатель/3(Ускорение) -> wd/1
  thetaRef/1 -> Заданный угол/1

== system hexapod2/Hexapod/Leg6/Servo2 ==
  note: ThetaRef
  note: e
  note: Vref
  thetaRef : Inport
  PID : Subsystem
  Sum : Sum  Inputs=|+-
  Thet : Scope
      settings: TimeRange=10  YMin=0  YMax=21
  w : Scope
      settings: SaveName=ScopeData2
  wd : Scope
      settings: SaveName=ScopeData3
  Двигатель : Subsystem
  Заданный угол : Gain
  Энкодер : Gain  Gain=Ke
  theta : Outport
  wires:
  thetaRef/1 -> Заданный угол/1
  Двигатель/3(Ускорение) -> wd/1
  PID/1(Out1) -> Двигатель/1(Заданный угол)
  Двигатель/1(Угол) -> Энкодер/1, Thet/1, theta/1
  Энкодер/1 -> Sum/2
  Sum/1 -> PID/1(In1)
  Заданный угол/1 -> Sum/1
  Двигатель/2(Скорость) -> w/1

== system hexapod2/Forward Kinematic/Create TGb/Switch1/t <= 5 ==
  Clock : Clock
  Constant : Constant  Value=3
  Relational Operator : RelationalOperator  Operator=<=  InputSameDT=on
  t <= 3 : Outport  InitialOutput=0
  wires:
  Relational Operator/1 -> t <= 3/1
  Clock/1 -> Relational Operator/1
  Constant/1 -> Relational Operator/2

== system hexapod2/Forward Kinematic/Create TGb/Switch2/t <= 1 ==
  Clock : Clock
  Constant : Constant  Value=3
  Relational Operator : RelationalOperator  Operator=<=  InputSameDT=on
  t <= 3 : Outport  InitialOutput=0
  wires:
  Constant/1 -> Relational Operator/2
  Clock/1 -> Relational Operator/1
  Relational Operator/1 -> t <= 3/1

== system hexapod2/Hexapod/Leg1/Servo/PID ==
  In1 : Inport
  Derivative : Derivative
  Integrator : Integrator
  Kp : Gain  Gain=64
  Kp1 : Gain  Gain=3.4
  Kp2 : Gain  Gain=0
  Sum : Sum  Inputs=|+++
  Out1 : Outport
  wires:
  In1/1 -> Kp2/1, Kp1/1, Kp/1
  Kp1/1 -> Derivative/1
  Sum/1 -> Out1/1
  Kp2/1 -> Integrator/1
  Integrator/1 -> Sum/1
  Kp/1 -> Sum/2
  Derivative/1 -> Sum/3

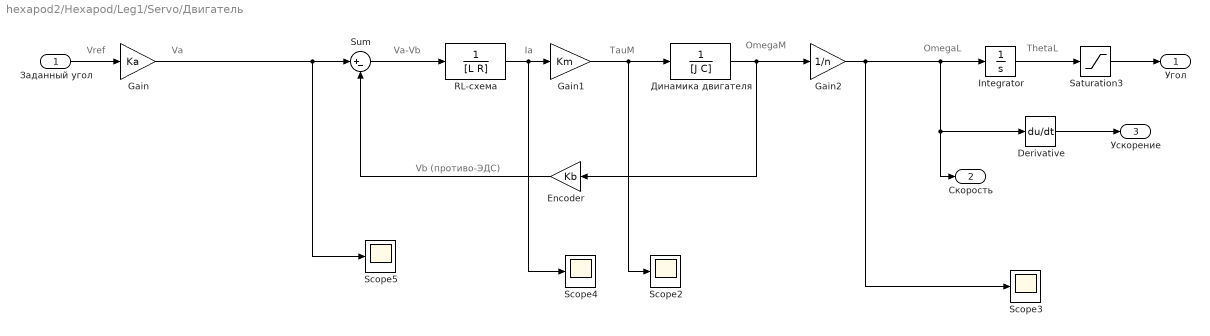
== system hexapod2/Hexapod/Leg1/Servo/Двигатель ==
  note: ThetaL
  note: OmegaL
  note: OmegaM
  note: TauM
  note: Ia
  note: Vb (противо-ЭДС)
  note: Va-Vb
  note: Va
  note: Vref
  Заданный угол : Inport
  Derivative : Derivative
  Encoder : Gain  Gain=Kb
  Gain : Gain  Gain=Ka
  Gain1 : Gain  Gain=Km
  Gain2 : Gain  Gain=1/n
  Integrator : Integrator
  RL-схема : TransferFcn  Denominator=[L R]
  Saturation3 : Saturate  UpperLimit=90*pi/180  LowerLimit=-90*pi/180  OutMin=[-150*pi/180]  OutMax=[150*pi/180]
  Scope{2..5} (4 alike) : Scope
      Scope3 settings: SaveName=ScopeData4
      Scope4 settings: SaveName=ScopeData5
      Scope5 settings: SaveName=ScopeData6
  Sum : Sum  Inputs=|+-
  Динамика двигателя : TransferFcn  Denominator=[J C]
  Угол : Outport
  Скорость : Outport  Port=2
  Ускорение : Outport  Port=3
  wires:
  RL-схема/1 -> Scope4/1, Gain1/1
  Sum/1 -> RL-схема/1
  Gain1/1 -> Динамика двигателя/1, Scope2/1
  Encoder/1 -> Sum/2
  Динамика двигателя/1 -> Gain2/1, Encoder/1
  Integrator/1 -> Saturation3/1
  Заданный угол/1 -> Gain/1
  Gain2/1 -> Derivative/1, Скорость/1, Integrator/1, Scope3/1
  Gain/1 -> Scope5/1, Sum/1
  Saturation3/1 -> Угол/1
  Derivative/1 -> Ускорение/1

== system hexapod2/Hexapod/Leg1/Servo1/PID ==
  In1 : Inport
  Derivative : Derivative
  Integrator : Integrator
  Kp : Gain  Gain=64
  Kp1 : Gain  Gain=3.4
  Kp2 : Gain  Gain=0
  Sum : Sum  Inputs=|+++
  Out1 : Outport
  wires:
  Derivative/1 -> Sum/3
  Kp/1 -> Sum/2
  Integrator/1 -> Sum/1
  Kp2/1 -> Integrator/1
  Sum/1 -> Out1/1
  Kp1/1 -> Derivative/1
  In1/1 -> Kp/1, Kp1/1, Kp2/1

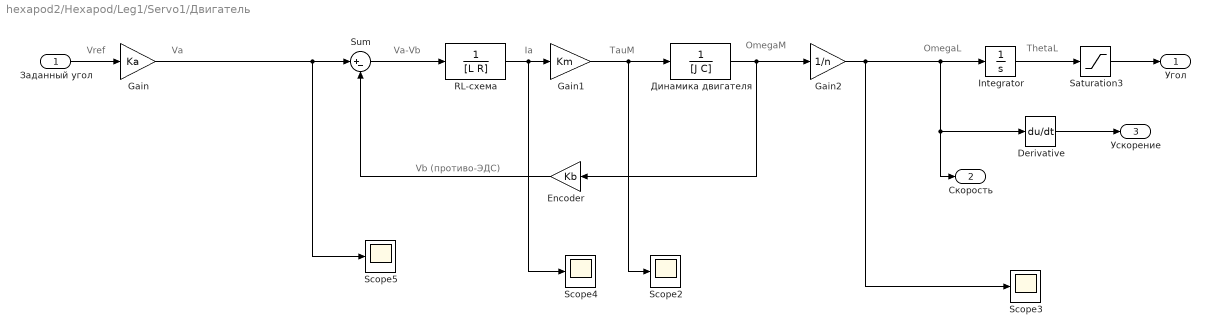
== system hexapod2/Hexapod/Leg1/Servo1/Двигатель ==
  note: Vref
  note: Va
  note: Va-Vb
  note: Vb (противо-ЭДС)
  note: Ia
  note: TauM
  note: OmegaM
  note: OmegaL
  note: ThetaL
  Заданный угол : Inport
  Derivative : Derivative
  Encoder : Gain  Gain=Kb
  Gain : Gain  Gain=Ka
  Gain1 : Gain  Gain=Km
  Gain2 : Gain  Gain=1/n
  Integrator : Integrator
  RL-схема : TransferFcn  Denominator=[L R]
  Saturation3 : Saturate  UpperLimit=90*pi/180  LowerLimit=-90*pi/180  OutMin=[-150*pi/180]  OutMax=[150*pi/180]
  Scope{2..5} (4 alike) : Scope
      Scope3 settings: SaveName=ScopeData4
      Scope4 settings: SaveName=ScopeData5
      Scope5 settings: SaveName=ScopeData6
  Sum : Sum  Inputs=|+-
  Динамика двигателя : TransferFcn  Denominator=[J C]
  Угол : Outport
  Скорость : Outport  Port=2
  Ускорение : Outport  Port=3
  wires:
  Derivative/1 -> Ускорение/1
  Saturation3/1 -> Угол/1
  Gain/1 -> Sum/1, Scope5/1
  Gain2/1 -> Scope3/1, Integrator/1, Скорость/1, Derivative/1
  Заданный угол/1 -> Gain/1
  Integrator/1 -> Saturation3/1
  Динамика двигателя/1 -> Encoder/1, Gain2/1
  Encoder/1 -> Sum/2
  Gain1/1 -> Scope2/1, Динамика двигателя/1
  Sum/1 -> RL-схема/1
  RL-схема/1 -> Gain1/1, Scope4/1

== system hexapod2/Hexapod/Leg1/Servo2/PID ==
  In1 : Inport
  Derivative : Derivative
  Integrator : Integrator
  Kp : Gain  Gain=64
  Kp1 : Gain  Gain=3.4
  Kp2 : Gain  Gain=0
  Sum : Sum  Inputs=|+++
  Out1 : Outport
  wires:
  In1/1 -> Kp2/1, Kp1/1, Kp/1
  Kp1/1 -> Derivative/1
  Sum/1 -> Out1/1
  Kp2/1 -> Integrator/1
  Integrator/1 -> Sum/1
  Kp/1 -> Sum/2
  Derivative/1 -> Sum/3

== system hexapod2/Hexapod/Leg1/Servo2/Двигатель ==
  note: ThetaL
  note: OmegaL
  note: OmegaM
  note: TauM
  note: Ia
  note: Vb (противо-ЭДС)
  note: Va-Vb
  note: Va
  note: Vref
  Заданный угол : Inport
  Derivative : Derivative
  Encoder : Gain  Gain=Kb
  Gain : Gain  Gain=Ka
  Gain1 : Gain  Gain=Km
  Gain2 : Gain  Gain=1/n
  Integrator : Integrator
  RL-схема : TransferFcn  Denominator=[L R]
  Saturation3 : Saturate  UpperLimit=90*pi/180  LowerLimit=-90*pi/180  OutMin=[-150*pi/180]  OutMax=[150*pi/180]
  Scope{2..5} (4 alike) : Scope
      Scope3 settings: SaveName=ScopeData4
      Scope4 settings: SaveName=ScopeData5
      Scope5 settings: SaveName=ScopeData6
  Sum : Sum  Inputs=|+-
  Динамика двигателя : TransferFcn  Denominator=[J C]
  Угол : Outport
  Скорость : Outport  Port=2
  Ускорение : Outport  Port=3
  wires:
  RL-схема/1 -> Scope4/1, Gain1/1
  Sum/1 -> RL-схема/1
  Gain1/1 -> Динамика двигателя/1, Scope2/1
  Encoder/1 -> Sum/2
  Динамика двигателя/1 -> Gain2/1, Encoder/1
  Integrator/1 -> Saturation3/1
  Заданный угол/1 -> Gain/1
  Gain2/1 -> Derivative/1, Скорость/1, Integrator/1, Scope3/1
  Gain/1 -> Scope5/1, Sum/1
  Saturation3/1 -> Угол/1
  Derivative/1 -> Ускорение/1

== system hexapod2/Hexapod/Leg2/Servo/PID ==
  In1 : Inport
  Derivative : Derivative
  Integrator : Integrator
  Kp : Gain  Gain=64
  Kp1 : Gain  Gain=3.4
  Kp2 : Gain  Gain=0
  Sum : Sum  Inputs=|+++
  Out1 : Outport
  wires:
  Derivative/1 -> Sum/3
  Kp/1 -> Sum/2
  Integrator/1 -> Sum/1
  Kp2/1 -> Integrator/1
  Sum/1 -> Out1/1
  Kp1/1 -> Derivative/1
  In1/1 -> Kp/1, Kp1/1, Kp2/1

== system hexapod2/Hexapod/Leg2/Servo/Двигатель ==
  note: Vref
  note: Va
  note: Va-Vb
  note: Vb (противо-ЭДС)
  note: Ia
  note: TauM
  note: OmegaM
  note: OmegaL
  note: ThetaL
  Заданный угол : Inport
  Derivative : Derivative
  Encoder : Gain  Gain=Kb
  Gain : Gain  Gain=Ka
  Gain1 : Gain  Gain=Km
  Gain2 : Gain  Gain=1/n
  Integrator : Integrator
  RL-схема : TransferFcn  Denominator=[L R]
  Saturation3 : Saturate  UpperLimit=90*pi/180  LowerLimit=-90*pi/180  OutMin=[-150*pi/180]  OutMax=[150*pi/180]
  Scope{2..5} (4 alike) : Scope
      Scope3 settings: SaveName=ScopeData4
      Scope4 settings: SaveName=ScopeData5
      Scope5 settings: SaveName=ScopeData6
  Sum : Sum  Inputs=|+-
  Динамика двигателя : TransferFcn  Denominator=[J C]
  Угол : Outport
  Скорость : Outport  Port=2
  Ускорение : Outport  Port=3
  wires:
  Derivative/1 -> Ускорение/1
  Saturation3/1 -> Угол/1
  Gain/1 -> Sum/1, Scope5/1
  Gain2/1 -> Scope3/1, Integrator/1, Скорость/1, Derivative/1
  Заданный угол/1 -> Gain/1
  Integrator/1 -> Saturation3/1
  Динамика двигателя/1 -> Encoder/1, Gain2/1
  Encoder/1 -> Sum/2
  Gain1/1 -> Scope2/1, Динамика двигателя/1
  Sum/1 -> RL-схема/1
  RL-схема/1 -> Gain1/1, Scope4/1

== system hexapod2/Hexapod/Leg2/Servo1/PID ==
  In1 : Inport
  Derivative : Derivative
  Integrator : Integrator
  Kp : Gain  Gain=64
  Kp1 : Gain  Gain=3.4
  Kp2 : Gain  Gain=0
  Sum : Sum  Inputs=|+++
  Out1 : Outport
  wires:
  In1/1 -> Kp2/1, Kp1/1, Kp/1
  Kp1/1 -> Derivative/1
  Sum/1 -> Out1/1
  Kp2/1 -> Integrator/1
  Integrator/1 -> Sum/1
  Kp/1 -> Sum/2
  Derivative/1 -> Sum/3

== system hexapod2/Hexapod/Leg2/Servo1/Двигатель ==
  note: ThetaL
  note: OmegaL
  note: OmegaM
  note: TauM
  note: Ia
  note: Vb (противо-ЭДС)
  note: Va-Vb
  note: Va
  note: Vref
  Заданный угол : Inport
  Derivative : Derivative
  Encoder : Gain  Gain=Kb
  Gain : Gain  Gain=Ka
  Gain1 : Gain  Gain=Km
  Gain2 : Gain  Gain=1/n
  Integrator : Integrator
  RL-схема : TransferFcn  Denominator=[L R]
  Saturation3 : Saturate  UpperLimit=90*pi/180  LowerLimit=-90*pi/180  OutMin=[-150*pi/180]  OutMax=[150*pi/180]
  Scope{2..5} (4 alike) : Scope
      Scope3 settings: SaveName=ScopeData4
      Scope4 settings: SaveName=ScopeData5
      Scope5 settings: SaveName=ScopeData6
  Sum : Sum  Inputs=|+-
  Динамика двигателя : TransferFcn  Denominator=[J C]
  Угол : Outport
  Скорость : Outport  Port=2
  Ускорение : Outport  Port=3
  wires:
  RL-схема/1 -> Scope4/1, Gain1/1
  Sum/1 -> RL-схема/1
  Gain1/1 -> Динамика двигателя/1, Scope2/1
  Encoder/1 -> Sum/2
  Динамика двигателя/1 -> Gain2/1, Encoder/1
  Integrator/1 -> Saturation3/1
  Заданный угол/1 -> Gain/1
  Gain2/1 -> Derivative/1, Скорость/1, Integrator/1, Scope3/1
  Gain/1 -> Scope5/1, Sum/1
  Saturation3/1 -> Угол/1
  Derivative/1 -> Ускорение/1

== system hexapod2/Hexapod/Leg2/Servo2/PID ==
  In1 : Inport
  Derivative : Derivative
  Integrator : Integrator
  Kp : Gain  Gain=64
  Kp1 : Gain  Gain=3.4
  Kp2 : Gain  Gain=0
  Sum : Sum  Inputs=|+++
  Out1 : Outport
  wires:
  Derivative/1 -> Sum/3
  Kp/1 -> Sum/2
  Integrator/1 -> Sum/1
  Kp2/1 -> Integrator/1
  Sum/1 -> Out1/1
  Kp1/1 -> Derivative/1
  In1/1 -> Kp/1, Kp1/1, Kp2/1

== system hexapod2/Hexapod/Leg2/Servo2/Двигатель ==
  note: Vref
  note: Va
  note: Va-Vb
  note: Vb (противо-ЭДС)
  note: Ia
  note: TauM
  note: OmegaM
  note: OmegaL
  note: ThetaL
  Заданный угол : Inport
  Derivative : Derivative
  Encoder : Gain  Gain=Kb
  Gain : Gain  Gain=Ka
  Gain1 : Gain  Gain=Km
  Gain2 : Gain  Gain=1/n
  Integrator : Integrator
  RL-схема : TransferFcn  Denominator=[L R]
  Saturation3 : Saturate  UpperLimit=90*pi/180  LowerLimit=-90*pi/180  OutMin=[-150*pi/180]  OutMax=[150*pi/180]
  Scope{2..5} (4 alike) : Scope
      Scope3 settings: SaveName=ScopeData4
      Scope4 settings: SaveName=ScopeData5
      Scope5 settings: SaveName=ScopeData6
  Sum : Sum  Inputs=|+-
  Динамика двигателя : TransferFcn  Denominator=[J C]
  Угол : Outport
  Скорость : Outport  Port=2
  Ускорение : Outport  Port=3
  wires:
  Derivative/1 -> Ускорение/1
  Saturation3/1 -> Угол/1
  Gain/1 -> Sum/1, Scope5/1
  Gain2/1 -> Scope3/1, Integrator/1, Скорость/1, Derivative/1
  Заданный угол/1 -> Gain/1
  Integrator/1 -> Saturation3/1
  Динамика двигателя/1 -> Encoder/1, Gain2/1
  Encoder/1 -> Sum/2
  Gain1/1 -> Scope2/1, Динамика двигателя/1
  Sum/1 -> RL-схема/1
  RL-схема/1 -> Gain1/1, Scope4/1

== system hexapod2/Hexapod/Leg3/Servo/PID ==
  In1 : Inport
  Derivative : Derivative
  Integrator : Integrator
  Kp : Gain  Gain=64
  Kp1 : Gain  Gain=3.4
  Kp2 : Gain  Gain=0
  Sum : Sum  Inputs=|+++
  Out1 : Outport
  wires:
  In1/1 -> Kp2/1, Kp1/1, Kp/1
  Kp1/1 -> Derivative/1
  Sum/1 -> Out1/1
  Kp2/1 -> Integrator/1
  Integrator/1 -> Sum/1
  Kp/1 -> Sum/2
  Derivative/1 -> Sum/3

== system hexapod2/Hexapod/Leg3/Servo/Двигатель ==
  note: ThetaL
  note: OmegaL
  note: OmegaM
  note: TauM
  note: Ia
  note: Vb (противо-ЭДС)
  note: Va-Vb
  note: Va
  note: Vref
  Заданный угол : Inport
  Derivative : Derivative
  Encoder : Gain  Gain=Kb
  Gain : Gain  Gain=Ka
  Gain1 : Gain  Gain=Km
  Gain2 : Gain  Gain=1/n
  Integrator : Integrator
  RL-схема : TransferFcn  Denominator=[L R]
  Saturation3 : Saturate  UpperLimit=90*pi/180  LowerLimit=-90*pi/180  OutMin=[-150*pi/180]  OutMax=[150*pi/180]
  Scope{2..5} (4 alike) : Scope
      Scope3 settings: SaveName=ScopeData4
      Scope4 settings: SaveName=ScopeData5
      Scope5 settings: SaveName=ScopeData6
  Sum : Sum  Inputs=|+-
  Динамика двигателя : TransferFcn  Denominator=[J C]
  Угол : Outport
  Скорость : Outport  Port=2
  Ускорение : Outport  Port=3
  wires:
  RL-схема/1 -> Scope4/1, Gain1/1
  Sum/1 -> RL-схема/1
  Gain1/1 -> Динамика двигателя/1, Scope2/1
  Encoder/1 -> Sum/2
  Динамика двигателя/1 -> Gain2/1, Encoder/1
  Integrator/1 -> Saturation3/1
  Заданный угол/1 -> Gain/1
  Gain2/1 -> Derivative/1, Скорость/1, Integrator/1, Scope3/1
  Gain/1 -> Scope5/1, Sum/1
  Saturation3/1 -> Угол/1
  Derivative/1 -> Ускорение/1

== system hexapod2/Hexapod/Leg3/Servo1/PID ==
  In1 : Inport
  Derivative : Derivative
  Integrator : Integrator
  Kp : Gain  Gain=64
  Kp1 : Gain  Gain=3.4
  Kp2 : Gain  Gain=0
  Sum : Sum  Inputs=|+++
  Out1 : Outport
  wires:
  Derivative/1 -> Sum/3
  Kp/1 -> Sum/2
  Integrator/1 -> Sum/1
  Kp2/1 -> Integrator/1
  Sum/1 -> Out1/1
  Kp1/1 -> Derivative/1
  In1/1 -> Kp/1, Kp1/1, Kp2/1

== system hexapod2/Hexapod/Leg3/Servo1/Двигатель ==
  note: Vref
  note: Va
  note: Va-Vb
  note: Vb (противо-ЭДС)
  note: Ia
  note: TauM
  note: OmegaM
  note: OmegaL
  note: ThetaL
  Заданный угол : Inport
  Derivative : Derivative
  Encoder : Gain  Gain=Kb
  Gain : Gain  Gain=Ka
  Gain1 : Gain  Gain=Km
  Gain2 : Gain  Gain=1/n
  Integrator : Integrator
  RL-схема : TransferFcn  Denominator=[L R]
  Saturation3 : Saturate  UpperLimit=90*pi/180  LowerLimit=-90*pi/180  OutMin=[-150*pi/180]  OutMax=[150*pi/180]
  Scope{2..5} (4 alike) : Scope
      Scope3 settings: SaveName=ScopeData4
      Scope4 settings: SaveName=ScopeData5
      Scope5 settings: SaveName=ScopeData6
  Sum : Sum  Inputs=|+-
  Динамика двигателя : TransferFcn  Denominator=[J C]
  Угол : Outport
  Скорость : Outport  Port=2
  Ускорение : Outport  Port=3
  wires:
  Derivative/1 -> Ускорение/1
  Saturation3/1 -> Угол/1
  Gain/1 -> Sum/1, Scope5/1
  Gain2/1 -> Scope3/1, Integrator/1, Скорость/1, Derivative/1
  Заданный угол/1 -> Gain/1
  Integrator/1 -> Saturation3/1
  Динамика двигателя/1 -> Encoder/1, Gain2/1
  Encoder/1 -> Sum/2
  Gain1/1 -> Scope2/1, Динамика двигателя/1
  Sum/1 -> RL-схема/1
  RL-схема/1 -> Gain1/1, Scope4/1

== system hexapod2/Hexapod/Leg3/Servo2/PID ==
  In1 : Inport
  Derivative : Derivative
  Integrator : Integrator
  Kp : Gain  Gain=64
  Kp1 : Gain  Gain=3.4
  Kp2 : Gain  Gain=0
  Sum : Sum  Inputs=|+++
  Out1 : Outport
  wires:
  In1/1 -> Kp2/1, Kp1/1, Kp/1
  Kp1/1 -> Derivative/1
  Sum/1 -> Out1/1
  Kp2/1 -> Integrator/1
  Integrator/1 -> Sum/1
  Kp/1 -> Sum/2
  Derivative/1 -> Sum/3

== system hexapod2/Hexapod/Leg3/Servo2/Двигатель ==
  note: ThetaL
  note: OmegaL
  note: OmegaM
  note: TauM
  note: Ia
  note: Vb (противо-ЭДС)
  note: Va-Vb
  note: Va
  note: Vref
  Заданный угол : Inport
  Derivative : Derivative
  Encoder : Gain  Gain=Kb
  Gain : Gain  Gain=Ka
  Gain1 : Gain  Gain=Km
  Gain2 : Gain  Gain=1/n
  Integrator : Integrator
  RL-схема : TransferFcn  Denominator=[L R]
  Saturation3 : Saturate  UpperLimit=90*pi/180  LowerLimit=-90*pi/180  OutMin=[-150*pi/180]  OutMax=[150*pi/180]
  Scope{2..5} (4 alike) : Scope
      Scope3 settings: SaveName=ScopeData4
      Scope4 settings: SaveName=ScopeData5
      Scope5 settings: SaveName=ScopeData6
  Sum : Sum  Inputs=|+-
  Динамика двигателя : TransferFcn  Denominator=[J C]
  Угол : Outport
  Скорость : Outport  Port=2
  Ускорение : Outport  Port=3
  wires:
  RL-схема/1 -> Scope4/1, Gain1/1
  Sum/1 -> RL-схема/1
  Gain1/1 -> Динамика двигателя/1, Scope2/1
  Encoder/1 -> Sum/2
  Динамика двигателя/1 -> Gain2/1, Encoder/1
  Integrator/1 -> Saturation3/1
  Заданный угол/1 -> Gain/1
  Gain2/1 -> Derivative/1, Скорость/1, Integrator/1, Scope3/1
  Gain/1 -> Scope5/1, Sum/1
  Saturation3/1 -> Угол/1
  Derivative/1 -> Ускорение/1

== system hexapod2/Hexapod/Leg4/Servo/PID ==
  In1 : Inport
  Derivative : Derivative
  Integrator : Integrator
  Kp : Gain  Gain=64
  Kp1 : Gain  Gain=3.4
  Kp2 : Gain  Gain=0
  Sum : Sum  Inputs=|+++
  Out1 : Outport
  wires:
  Derivative/1 -> Sum/3
  Kp/1 -> Sum/2
  Integrator/1 -> Sum/1
  Kp2/1 -> Integrator/1
  Sum/1 -> Out1/1
  Kp1/1 -> Derivative/1
  In1/1 -> Kp/1, Kp1/1, Kp2/1

== system hexapod2/Hexapod/Leg4/Servo/Двигатель ==
  note: Vref
  note: Va
  note: Va-Vb
  note: Vb (противо-ЭДС)
  note: Ia
  note: TauM
  note: OmegaM
  note: OmegaL
  note: ThetaL
  Заданный угол : Inport
  Derivative : Derivative
  Encoder : Gain  Gain=Kb
  Gain : Gain  Gain=Ka
  Gain1 : Gain  Gain=Km
  Gain2 : Gain  Gain=1/n
  Integrator : Integrator
  RL-схема : TransferFcn  Denominator=[L R]
  Saturation3 : Saturate  UpperLimit=90*pi/180  LowerLimit=-90*pi/180  OutMin=[-150*pi/180]  OutMax=[150*pi/180]
  Scope{2..5} (4 alike) : Scope
      Scope3 settings: SaveName=ScopeData4
      Scope4 settings: SaveName=ScopeData5
      Scope5 settings: SaveName=ScopeData6
  Sum : Sum  Inputs=|+-
  Динамика двигателя : TransferFcn  Denominator=[J C]
  Угол : Outport
  Скорость : Outport  Port=2
  Ускорение : Outport  Port=3
  wires:
  Derivative/1 -> Ускорение/1
  Saturation3/1 -> Угол/1
  Gain/1 -> Sum/1, Scope5/1
  Gain2/1 -> Scope3/1, Integrator/1, Скорость/1, Derivative/1
  Заданный угол/1 -> Gain/1
  Integrator/1 -> Saturation3/1
  Динамика двигателя/1 -> Encoder/1, Gain2/1
  Encoder/1 -> Sum/2
  Gain1/1 -> Scope2/1, Динамика двигателя/1
  Sum/1 -> RL-схема/1
  RL-схема/1 -> Gain1/1, Scope4/1

== system hexapod2/Hexapod/Leg4/Servo1/PID ==
  In1 : Inport
  Derivative : Derivative
  Integrator : Integrator
  Kp : Gain  Gain=64
  Kp1 : Gain  Gain=3.4
  Kp2 : Gain  Gain=0
  Sum : Sum  Inputs=|+++
  Out1 : Outport
  wires:
  In1/1 -> Kp2/1, Kp1/1, Kp/1
  Kp1/1 -> Derivative/1
  Sum/1 -> Out1/1
  Kp2/1 -> Integrator/1
  Integrator/1 -> Sum/1
  Kp/1 -> Sum/2
  Derivative/1 -> Sum/3

== system hexapod2/Hexapod/Leg4/Servo1/Двигатель ==
  note: ThetaL
  note: OmegaL
  note: OmegaM
  note: TauM
  note: Ia
  note: Vb (противо-ЭДС)
  note: Va-Vb
  note: Va
  note: Vref
  Заданный угол : Inport
  Derivative : Derivative
  Encoder : Gain  Gain=Kb
  Gain : Gain  Gain=Ka
  Gain1 : Gain  Gain=Km
  Gain2 : Gain  Gain=1/n
  Integrator : Integrator
  RL-схема : TransferFcn  Denominator=[L R]
  Saturation3 : Saturate  UpperLimit=90*pi/180  LowerLimit=-90*pi/180  OutMin=[-150*pi/180]  OutMax=[150*pi/180]
  Scope{2..5} (4 alike) : Scope
      Scope3 settings: SaveName=ScopeData4
      Scope4 settings: SaveName=ScopeData5
      Scope5 settings: SaveName=ScopeData6
  Sum : Sum  Inputs=|+-
  Динамика двигателя : TransferFcn  Denominator=[J C]
  Угол : Outport
  Скорость : Outport  Port=2
  Ускорение : Outport  Port=3
  wires:
  RL-схема/1 -> Scope4/1, Gain1/1
  Sum/1 -> RL-схема/1
  Gain1/1 -> Динамика двигателя/1, Scope2/1
  Encoder/1 -> Sum/2
  Динамика двигателя/1 -> Gain2/1, Encoder/1
  Integrator/1 -> Saturation3/1
  Заданный угол/1 -> Gain/1
  Gain2/1 -> Derivative/1, Скорость/1, Integrator/1, Scope3/1
  Gain/1 -> Scope5/1, Sum/1
  Saturation3/1 -> Угол/1
  Derivative/1 -> Ускорение/1

== system hexapod2/Hexapod/Leg4/Servo2/PID ==
  In1 : Inport
  Derivative : Derivative
  Integrator : Integrator
  Kp : Gain  Gain=64
  Kp1 : Gain  Gain=3.4
  Kp2 : Gain  Gain=0
  Sum : Sum  Inputs=|+++
  Out1 : Outport
  wires:
  Derivative/1 -> Sum/3
  Kp/1 -> Sum/2
  Integrator/1 -> Sum/1
  Kp2/1 -> Integrator/1
  Sum/1 -> Out1/1
  Kp1/1 -> Derivative/1
  In1/1 -> Kp/1, Kp1/1, Kp2/1

== system hexapod2/Hexapod/Leg4/Servo2/Двигатель ==
  note: Vref
  note: Va
  note: Va-Vb
  note: Vb (противо-ЭДС)
  note: Ia
  note: TauM
  note: OmegaM
  note: OmegaL
  note: ThetaL
  Заданный угол : Inport
  Derivative : Derivative
  Encoder : Gain  Gain=Kb
  Gain : Gain  Gain=Ka
  Gain1 : Gain  Gain=Km
  Gain2 : Gain  Gain=1/n
  Integrator : Integrator
  RL-схема : TransferFcn  Denominator=[L R]
  Saturation3 : Saturate  UpperLimit=90*pi/180  LowerLimit=-90*pi/180  OutMin=[-150*pi/180]  OutMax=[150*pi/180]
  Scope{2..5} (4 alike) : Scope
      Scope3 settings: SaveName=ScopeData4
      Scope4 settings: SaveName=ScopeData5
      Scope5 settings: SaveName=ScopeData6
  Sum : Sum  Inputs=|+-
  Динамика двигателя : TransferFcn  Denominator=[J C]
  Угол : Outport
  Скорость : Outport  Port=2
  Ускорение : Outport  Port=3
  wires:
  Derivative/1 -> Ускорение/1
  Saturation3/1 -> Угол/1
  Gain/1 -> Sum/1, Scope5/1
  Gain2/1 -> Scope3/1, Integrator/1, Скорость/1, Derivative/1
  Заданный угол/1 -> Gain/1
  Integrator/1 -> Saturation3/1
  Динамика двигателя/1 -> Encoder/1, Gain2/1
  Encoder/1 -> Sum/2
  Gain1/1 -> Scope2/1, Динамика двигателя/1
  Sum/1 -> RL-схема/1
  RL-схема/1 -> Gain1/1, Scope4/1

== system hexapod2/Hexapod/Leg5/Servo/PID ==
  In1 : Inport
  Derivative : Derivative
  Integrator : Integrator
  Kp : Gain  Gain=64
  Kp1 : Gain  Gain=3.4
  Kp2 : Gain  Gain=0
  Sum : Sum  Inputs=|+++
  Out1 : Outport
  wires:
  In1/1 -> Kp2/1, Kp1/1, Kp/1
  Kp1/1 -> Derivative/1
  Sum/1 -> Out1/1
  Kp2/1 -> Integrator/1
  Integrator/1 -> Sum/1
  Kp/1 -> Sum/2
  Derivative/1 -> Sum/3
